simulink model "PTB_ConventionalModel"  (R2024a)
settings: Solver=ode23tb  StartTime=0.0  StopTime=150  RelTol=1e-4  AbsTol=1e-6
model workspace (MAT data in the model file):
  Af = 4
  Cd = 0.3
  D = 0.322411602927
  DownShiftSpeeds = [11.05 18.7 28.9 38.675 51.425 11.05 18.7 28.9 38.675 51.425 11.05 18.7 ... (85 elements, 5x17)]
  DrCycles : object (value not decoded)
  I = 0.25
  Kbr = 10000
  P = 15
  PedalPositions = [0 6.2485 12.4969 18.7454 24.9939 31.2424 37.4908 43.7393 49.9878 56.2363 62.4847 68.7332 ... (17 elements, 1x17)]
  TimeHWFET = 765
  TimeUDDS = 1372
  TimeUS06 = 596
  UpShiftSpeeds = [12.75 20.997635 31.45 42.16136 55.58864 12.75 20.997635 31.45 42.16136 55.58864 12.75 20.997635 ... (85 elements, 5x17)]
  axle_b = 10
  axle_k = 5000
  convAxle_wc = 500
  diffRatio = 3.4
  driveshaft_b = 10
  driveshaft_k = 2500
  driveshaft_wc = 500
  engineSpeedPoints_rpm = [750 1053.57142857 1357.14285714 1660.71428571 1964.28571429 2267.85714286 2571.42857143 2875 3178.57142857 3482.14285714 3785.71428571 4089.28571429 ... (15 elements, 1x15)]
  engineTorqueMap_Nm = [-13.6738264269 15.0034460821 26.4289521305 37.8539339756 49.2854604964 60.7146317399 72.0173711595 77.7345012802 77.7345012802 77.7345012802 77.7345012802 77.7345012802 ... (240 elements, 16x15)]
  engineTorquePoints_Nm = [0 15 26.4285714286 37.8571428571 49.2857142857 60.7142857143 72.1428571429 83.5714285714 95 106.428571429 117.857142857 129.285714286 ... (16 elements, 1x16)]
  vehicleMass = 1500
  wheelRadius = 0.35
values from neighbouring files (symbols this model uses):
  m = 0:0.01:10    [acc_GA.m]
  s = tf('s')    [PIDTune_GeneticAlgorithm.m]    (also in pidtest.m; plots_GA.m; tf_acc_deneme.m)
libraries: Wheels_Driver_VehDyn_Lib x6, autolibsharedcoupling x4, simulink x4, autolibshareddiff x2, autolibsharedtransfixedgear x2, autolibsharedmappedengines x2, autolibshared x1, slpidlib x1
(part 3 of 5)

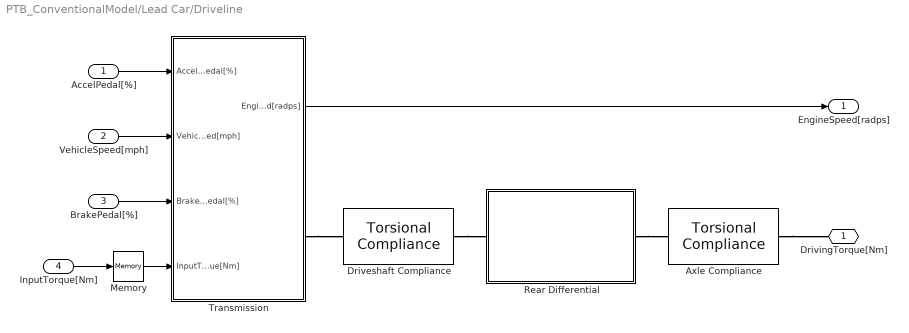
== system PTB_ConventionalModel/Lead Car/Driveline ==
  AccelPedal[%] : Inport
  VehicleSpeed[mph] : Inport  Port=2
  BrakePedal[%] : Inport  Port=3
  InputTorque[Nm] : Inport  Port=4
  Axle Compliance : autolibsharedcoupling/Torsional Compliance  port_config=Two-way connection  extInfo=off  k=axle_k  b=axle_b  theta_o=0  domega_o=0  omega_c=convAxle_wc  blkID=0  aMode=1
  Driveshaft Compliance : autolibsharedcoupling/Torsional Compliance  port_config=Two-way connection  extInfo=off  k=driveshaft_k  b=driveshaft_b  theta_o=0  domega_o=0  omega_c=driveshaft_wc  blkID=0  aMode=1
  Memory : Memory
  Rear Differential : Subsystem
  Transmission : Subsystem
  DrivingTorque[Nm] : PMIOPort  Side=Right
  EngineSpeed[radps] : Outport  VectorParamsAs1DForOutWhenUnconnected=off
  wires:
  Transmission/1(EngineSpeed[radps]) -> EngineSpeed[radps]/1
  InputTorque[Nm]/1 -> Memory/1
  AccelPedal[%]/1 -> Transmission/1(AccelPedal[%])
  VehicleSpeed[mph]/1 -> Transmission/2(VehicleSpeed[mph])
  BrakePedal[%]/1 -> Transmission/3(BrakePedal[%])
  Memory/1 -> Transmission/4(InputTorque[Nm])
  connections:
  Axle Compliance/RConn1 -- DrivingTorque[Nm]/RConn1
  Rear Differential/RConn1 -- Axle Compliance/LConn1
  Driveshaft Compliance/RConn1 -- Rear Differential/LConn1
  Transmission/RConn1 -- Driveshaft Compliance/LConn1
